simulink model "error_stable_state"  (R2015a)
settings: Solver=ode45  StartTime=0.0  StopTime=5000  RelTol=1e-3
libraries: simulink x6
settings Model: Creator=Jose Roldan  LastModifiedBy=Jose Roldan

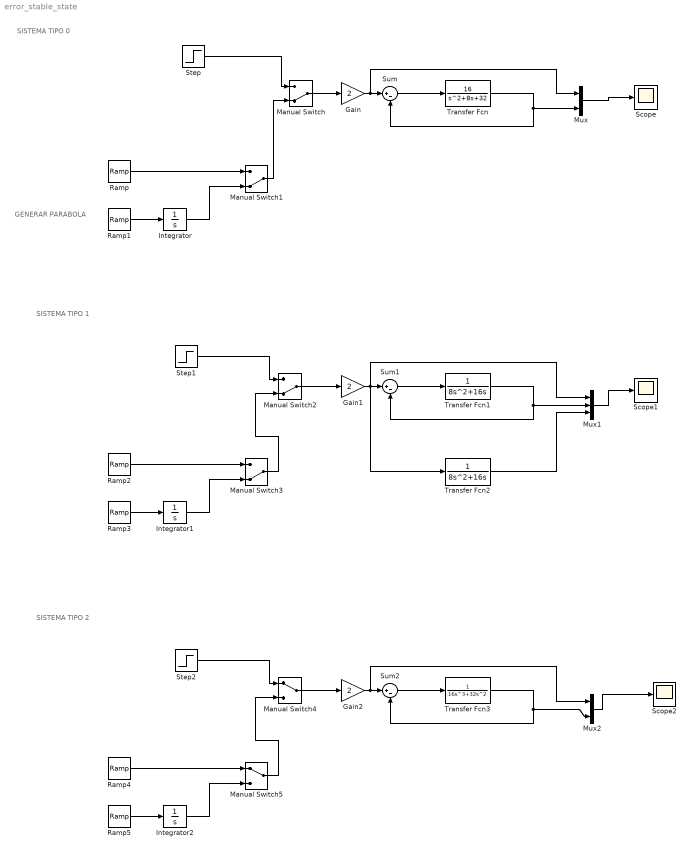
== system error_stable_state ==
  note: SISTEMA TIPO 1
  note: SISTEMA TIPO 0
  note: GENERAR PARABOLA
  note: SISTEMA TIPO 2
  Gain : Gain  Gain=2
  Gain1 : Gain  Gain=2
  Gain2 : Gain  Gain=2
  Integrator : Integrator
  Integrator1 : Integrator
  Integrator2 : Integrator
  Manual Switch{,1..3} (4 alike) : ManualSwitch  CurrentSetting=0
  Manual Switch4 : ManualSwitch
  Manual Switch5 : ManualSwitch
  Mux : Mux  Inputs=2
  Mux1 : Mux  Inputs=3
  Mux2 : Mux  Inputs=2
  Ramp{,1..5} (6 alike) : simulink/Sources/Ramp  slope=1  start=0  X0=0
  Scope : Scope
  Scope1 : Scope
  Scope2 : Scope
      settings: SaveName=ScopeData2
  Step : Step  SampleTime=0
  Step1 : Step  SampleTime=0
  Step2 : Step  SampleTime=0
  Sum : Sum  Inputs=|+-
  Sum1 : Sum  Inputs=|+-
  Sum2 : Sum  Inputs=|+-
  Transfer Fcn : TransferFcn  Numerator=[16]  Denominator=[1 8 32]
  Transfer Fcn1 : TransferFcn  Denominator=[8 16 0]
  Transfer Fcn2 : TransferFcn  Denominator=[8 16 0]
  Transfer Fcn3 : TransferFcn  Denominator=[16 32 0 0]
  wires:
  Sum/1 -> Transfer Fcn/1
  Transfer Fcn/1 -> Mux/2, Sum/2
  Mux/1 -> Scope/1
  Step/1 -> Manual Switch/1
  Ramp1/1 -> Integrator/1
  Ramp/1 -> Manual Switch1/1
  Integrator/1 -> Manual Switch1/2
  Manual Switch1/1 -> Manual Switch/2
  Manual Switch/1 -> Gain/1
  Gain/1 -> Mux/1, Sum/1
  Sum1/1 -> Transfer Fcn1/1
  Transfer Fcn1/1 -> Mux1/2, Sum1/2
  Mux1/1 -> Scope1/1
  Step1/1 -> Manual Switch2/1
  Ramp3/1 -> Integrator1/1
  Ramp2/1 -> Manual Switch3/1
  Integrator1/1 -> Manual Switch3/2
  Manual Switch3/1 -> Manual Switch2/2
  Manual Switch2/1 -> Gain1/1
  Gain1/1 -> Transfer Fcn2/1, Mux1/1, Sum1/1
  Transfer Fcn2/1 -> Mux1/3
  Sum2/1 -> Transfer Fcn3/1
  Transfer Fcn3/1 -> Mux2/2, Sum2/2
  Mux2/1 -> Scope2/1
  Step2/1 -> Manual Switch4/1
  Ramp5/1 -> Integrator2/1
  Ramp4/1 -> Manual Switch5/1
  Integrator2/1 -> Manual Switch5/2
  Manual Switch5/1 -> Manual Switch4/2
  Manual Switch4/1 -> Gain2/1
  Gain2/1 -> Mux2/1, Sum2/1
